simulink model "phase1_delay_test"  (R2026a)
settings: Solver=ode4  StopTime=0.25  FixedStep=0.01
undefined symbols (not defined in the file or in its folder): test_delay_s
settings Model: Creator=rayyu  LastModifiedBy=rayyu

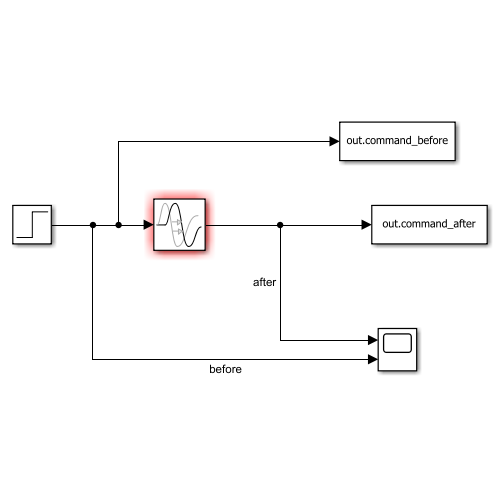
[thumbnail: Simulink's stored preview of the top-level diagram]
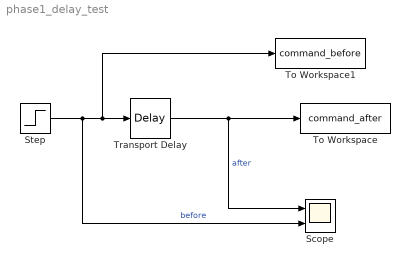
== system phase1_delay_test ==
  Scope : Scope  NumInputPorts=2
      settings: ActiveDisplayYMinimum=-0.4138864371338481  ActiveDisplayYMaximum=0.96416845840375909
  Step : Step  Time=0.01  SampleTime=0
  To Workspace : ToWorkspace  VariableName=command_after  SaveFormat=Timeseries  SampleTime=-1
  To Workspace1 : ToWorkspace  VariableName=command_before  SaveFormat=Timeseries  SampleTime=-1
  Transport Delay : TransportDelay  DelayTime=test_delay_s
  wires:
  Step/1 -> Scope/2, To Workspace1/1, Transport Delay/1  "before"
  Transport Delay/1 -> Scope/1, To Workspace/1  "after"
